simulink model "SchemaBlocSimulink"  (R2015a)
settings: Solver=ode45  StartTime=0.0  StopTime=10.0  RelTol=1e-3
undefined symbols (not defined in the file or in its folder): denF1, denF2, denF3, denF4, numF1, numF2, numF3, numF4
settings Model: Creator=Utilisateur  LastModifiedBy=Utilisateur
settings SolverCC: AlgebraicLoopSolver=LineSearch

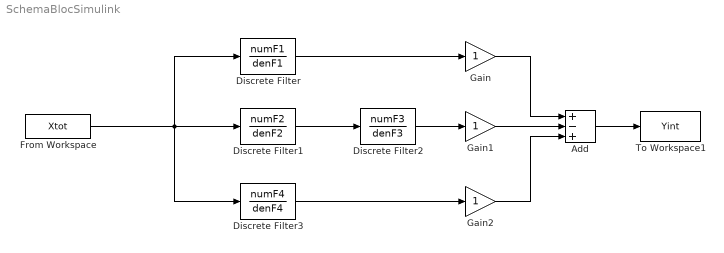
== system SchemaBlocSimulink ==
  Add : Sum  Inputs=+-+
  Discrete Filter : DiscreteFilter  Numerator=numF1  Denominator=denF1  InputProcessing=Columns as channels (frame based)  FilterStructure=Direct form I  SampleTime=44100
  Discrete Filter1 : DiscreteFilter  Numerator=numF2  Denominator=denF2  InputProcessing=Columns as channels (frame based)  FilterStructure=Direct form I  SampleTime=44100
  Discrete Filter2 : DiscreteFilter  Numerator=numF3  Denominator=denF3  InputProcessing=Columns as channels (frame based)  FilterStructure=Direct form I  SampleTime=44100
  Discrete Filter3 : DiscreteFilter  Numerator=numF4  Denominator=denF4  InputProcessing=Columns as channels (frame based)  FilterStructure=Direct form I  SampleTime=44100
  From Workspace : FromWorkspace  VariableName=Xtot  SampleTime=1
  Gain : Gain
  Gain1 : Gain
  Gain2 : Gain
  To Workspace1 : ToWorkspace  VariableName=Yint  SampleTime=-1
  wires:
  From Workspace/1 -> Discrete Filter/1, Discrete Filter3/1, Discrete Filter1/1
  Discrete Filter/1 -> Gain/1
  Gain/1 -> Add/1
  Gain1/1 -> Add/2
  Gain2/1 -> Add/3
  Add/1 -> To Workspace1/1
  Discrete Filter3/1 -> Gain2/1
  Discrete Filter2/1 -> Gain1/1
  Discrete Filter1/1 -> Discrete Filter2/1
